simulink model "udpRead"  (R2015b)
settings: Solver=FixedStepDiscrete  StartTime=0.0  StopTime=inf  FixedStep=1/1000  RelTol=1e-3
libraries: simulink x3, embdlinuxlib x1
settings Model: SimulationMode=external  ExtModeEnableFloating=off  ExtModeTrigDuration=100  Creator=Nik Descher  LastModifiedBy=Nik Descher
settings DataIOCC: LimitDataPoints=off
settings OptimizationCC: OptimizeModelRefInitCode=on  LifeSpan=1
settings HardwareCC: ProdBitPerPointer=32  ProdLargestAtomicInteger=Long  ProdLargestAtomicFloat=Double  ProdWordSize=32  ProdHWDeviceType=ARM Compatible->ARM Cortex
settings RTWCC: SystemTargetFile=realtime.tlc  GenerateMakefile=off  TemplateMakefile=realtime.tmf  Description=Run on Target Hardware  RTWVerbose=off
settings STFCustomTargetCC: TargetLibSuffix=.a  GenerateSampleERTMain=on  ConcurrentExecutionCompliant=off  GeneratePreprocessorConditionals=Use local settings  ERTCustomFileBanners=on  SupportNonInlinedSFcns=off  SupportVariableSizeSignals=on  MATLABClassNameForMDSCustomization=Simulink.SoftwareTarget.ERTCustomization  CPPClassGenCompliant=off  GRTInterface=off  SystemTargetFile=realtime.tlc
settings ERTTargetCC: GenerateSampleERTMain=on  ParMdlRefBuildCompliant=off  CompOptLevelCompliant=off  ConcurrentExecutionCompliant=off  CombineOutputUpdateFcns=off  ERTFirstTimeCompliant=off  SupportContinuousTime=on  SupportVariableSizeSignals=on  ModelStepFunctionPrototypeControlCompliant=off  CPPClassGenCompliant=off  UseToolchainInfoCompliant=off  ExtModeMexArgs='192.168.1.248' 0 17724  ERTSrcFileBannerTemplate=realtime_code_template.cgt  ERTHdrFileBannerTemplate=realtime_code_template.cgt  ERTDataSrcFileTemplate=realtime_code_template.cgt  ERTDataHdrFileTemplate=realtime_code_template.cgt  ERTCustomFileTemplate=realtime_file_process.tlc

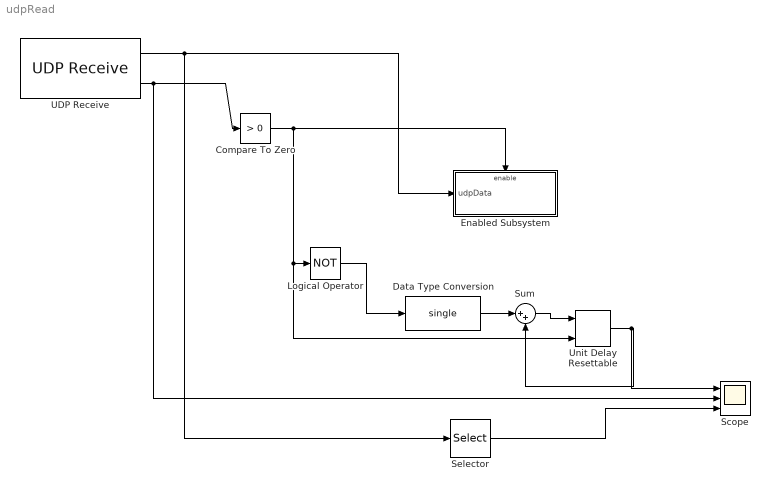
== system udpRead ==
  Compare To Zero : simulink/Logic and Bit Operations/Compare To Zero  relop=>  OutDataTypeStr=boolean
  Data Type Conversion : DataTypeConversion  OutDataTypeStr=single
  Enabled Subsystem : Subsystem  TreatAsAtomicUnit=on
  Logical Operator : Logic  Operator=NOT  AllPortsSameDT=off  OutDataTypeStr=boolean
  Scope : Scope  NumInputPorts=3
  Selector : Selector  InputPortWidth=31  IndexOptions=Index vector (dialog)  Indices=31  OutputSizes=1
  Sum : Sum  Inputs=|++
  UDP Receive : embdlinuxlib/UDP Receive  localURL='0.0.0.0'  localPort=25000  remoteURL='0.0.0.0'  remotePort=-1  recvBufferSize=8192  signalDatatype=single  dims=31  isVarSize=off  showBlockingTime=off  blockingTime=0  sampletime=1/1000  blockPlatform=Raspberry Pi
  Unit Delay Resettable : simulink/Additional Math & Discrete/Additional Discrete/Unit Delay Resettable  vinit=0  tsamp=-1
  wires:
  UDP Receive/1 -> Selector/1, Enabled Subsystem/1(udpData)
  UDP Receive/2 -> Scope/2, Compare To Zero/1
  Compare To Zero/1 -> Unit Delay Resettable/2, Logical Operator/1, Enabled Subsystem/Enable
  Unit Delay Resettable/1 -> Scope/1, Sum/2
  Logical Operator/1 -> Data Type Conversion/1
  Sum/1 -> Unit Delay Resettable/1
  Data Type Conversion/1 -> Sum/1
  Selector/1 -> Scope/3

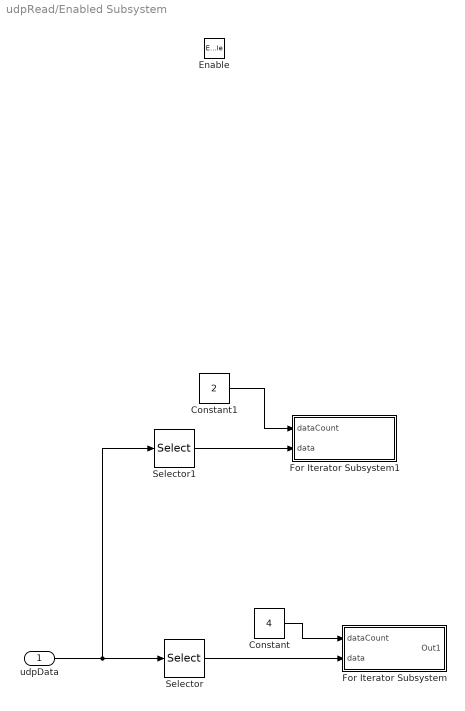
== system udpRead/Enabled Subsystem ==
  udpData : Inport
  Enable : EnablePort
  Constant : Constant  Value=4
  Constant1 : Constant  Value=2
  For Iterator Subsystem : Subsystem  TreatAsAtomicUnit=on
  For Iterator Subsystem1 : Subsystem  TreatAsAtomicUnit=on
  Selector : Selector  InputPortWidth=31  IndexOptions=Index vector (dialog)  Indices=1:24  OutputSizes=1
  Selector1 : Selector  InputPortWidth=31  IndexOptions=Index vector (dialog)  Indices=25:30  OutputSizes=1
  wires:
  udpData/1 -> Selector/1, Selector1/1
  Selector/1 -> For Iterator Subsystem/2(data)
  Constant/1 -> For Iterator Subsystem/1(dataCount)
  Selector1/1 -> For Iterator Subsystem1/2(data)
  Constant1/1 -> For Iterator Subsystem1/1(dataCount)

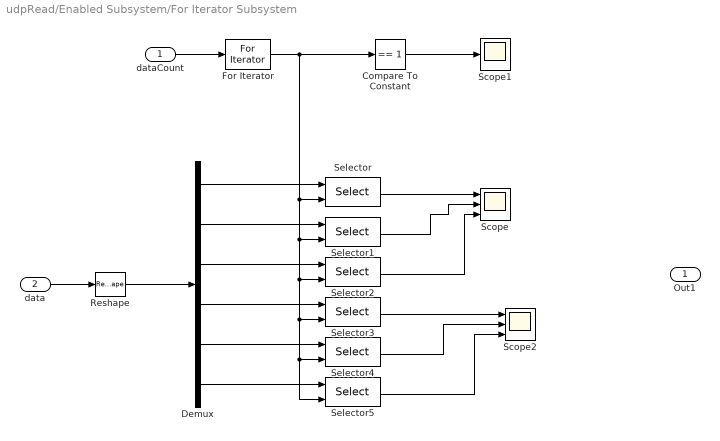
== system udpRead/Enabled Subsystem/For Iterator Subsystem ==
  dataCount : Inport
  data : Inport  Port=2
  Compare To Constant : simulink/Logic and Bit Operations/Compare To Constant  relop===  const=1  OutDataTypeStr=boolean
  Demux : Demux  Outputs=6
  For Iterator : ForIterator  IterationSource=external
  Reshape : Reshape
  Scope : Scope  NumInputPorts=3
  Scope1 : Scope
  Scope2 : Scope  NumInputPorts=3
  Selector{,1..5} (6 alike) : Selector  InputPortWidth=4  IndexOptions=Index vector (port)  Indices=[1 3]  OutputSizes=1
  Out1 : Outport
  wires:
  dataCount/1 -> For Iterator/1
  data/1 -> Reshape/1
  Demux/1 -> Selector/1
  For Iterator/1 -> Compare To Constant/1, Selector5/2, Selector4/2, Selector3/2, Selector2/2, Selector1/2, Selector/2
  Demux/2 -> Selector1/1
  Demux/3 -> Selector2/1
  Demux/4 -> Selector3/1
  Demux/5 -> Selector4/1
  Demux/6 -> Selector5/1
  Selector/1 -> Scope/1
  Selector1/1 -> Scope/2
  Selector2/1 -> Scope/3
  Compare To Constant/1 -> Scope1/1
  Reshape/1 -> Demux/1
  Selector3/1 -> Scope2/1
  Selector4/1 -> Scope2/2
  Selector5/1 -> Scope2/3

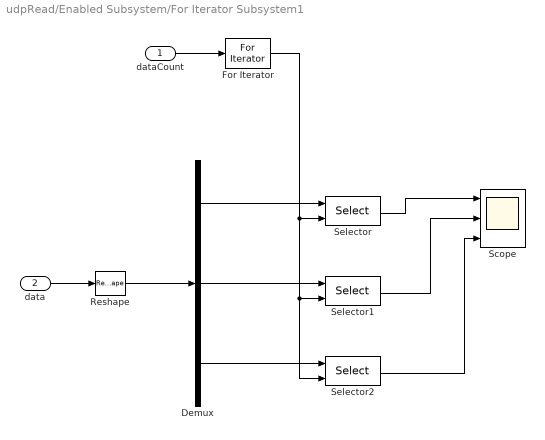
== system udpRead/Enabled Subsystem/For Iterator Subsystem1 ==
  dataCount : Inport
  data : Inport  Port=2
  Demux : Demux  Outputs=3
  For Iterator : ForIterator  IterationSource=external
  Reshape : Reshape
  Scope : Scope  NumInputPorts=3
  Selector : Selector  InputPortWidth=2  IndexOptions=Index vector (port)  Indices=[1 3]  OutputSizes=1
  Selector1 : Selector  InputPortWidth=2  IndexOptions=Index vector (port)  Indices=[1 3]  OutputSizes=1
  Selector2 : Selector  InputPortWidth=2  IndexOptions=Index vector (port)  Indices=[1 3]  OutputSizes=1
  wires:
  Reshape/1 -> Demux/1
  Selector2/1 -> Scope/3
  Selector1/1 -> Scope/2
  Selector/1 -> Scope/1
  Demux/3 -> Selector2/1
  Demux/2 -> Selector1/1
  For Iterator/1 -> Selector/2, Selector1/2, Selector2/2
  Demux/1 -> Selector/1
  data/1 -> Reshape/1
  dataCount/1 -> For Iterator/1
